simulink model "Main_simulation_optimised_accel_testbed"  (R2017b)
settings: Solver=FixedStepDiscrete  StartTime=0  StopTime=2474  RelTol=1e-3  EnableMultiTasking=on
PreLoadFcn:
  | Ts=2e-6;
undefined symbols (not defined in the file): Batt, BatteryCback, BatteryLoadFcn, DiscIntNeverNeededParam, Discrete, gcbh, Ion, Lithium, sigbuilder_block, sps_rtmsupport, spsBatteryModel
libraries: powerlib x53, electricdrivelib x6, simulink x6, autolibshared x6, powerlib_meascontrol x4, sdolib x3, spsDrivesDcBusModel x1, spsDrivesPrivateModels x1, spsDrivesOutputSelector x1, spsDrivesSpeedControllerModel x1
(part 2 of 3)

== system Main_simulation_optimised_accel_testbed/PMSM Drive vehicle ==
  Speed (rad/sec) : Inport
  Trq (Nm) : Inport  Port=2
  Bus Creator : BusCreator  Inputs=3
  Bus Selector : BusSelector  OutputSignals=V bus (V)
  DC_bus overvoltage protection : Subsystem  Commented=on
  PM Synchronous Motor Drive : Subsystem  DialogController=POWERSYS.PowerSysDialog  LoadFcn=|  mask(PM Synchronous Motor Drive){Rs=0.2, Lls=8.5e-3, Lms=8.5e-3, MachineConstant=Flux linkage established by magnets (V.s), FluxCst=0.175, VoltageCst=126.966, TorqueCst=1.05, ia=0, ib=0, J=0.089, Friction=0.005, p=4, wm=0, thetam=0, Rsnb_rec=10e3, Csnb_rec=20e-9, Ron_rec=1e-3, Vf_rec=1.3, cap_bus=200e-6, Rbrake=8, fbrake=4000, activationVoltage=190, shutdownVoltage=175, sourceFrequency=60, deviceType=IGBT / Diodes, Ron_inv=1e-3, Vf_inv=0.8, Vfd_inv=0.8, Tf=1e-6, Tt=2e-6, Tf_GTO=0, Tt_GTO=0, Rsnb_inv=5000, Csnb_inv=inf, regulationType=Speed regulation, Acc=1000, Dec=-1000, kp_sc=5, ki_sc=100, fc_sc=100, Tsc=7*20e-6, Tmin=-17.8, Tmax=17.8, modulationType=Hysteresis, h=0.1, kp_Id=200, ki_Id=1000, kp_Iq=200, ki_Iq=1000, fc_bus=50, car_freq=20000, freq_max=20e3, Tvect=20e-6, baseSampleTime=2e-06, outputBusMode=Multiple output buses, busLabels=off, MechanicalLoad=Torque Tm, modelDetailLevel=Detailed, driveType=AC6, AverageValue=off}
      | if ~isempty(get_param(gcb,'UserData')) 
      |       UserDataToSimulinkMask(gcbh,get_param(gcb,'driveType'));  
      |       set_param(gcb, 'UserData',[]);
      |       set_param(gcb,'UserDataPersistent','off');
      | end 
      | if strcmp(get_param(gcb,'AverageValue'),'on')
      |     set_param(gcb,'modelDetailLevel','Average');
      | end
      mask prompts: Rs "Resistance (ohm):"; Lls "D-axis inductance (H):"; Lms "Q-axis inductance (H):"; MachineConstant "Specify:"; ia "Phase A (A):"; ib "Phase B (A):"; J "Inertia (kg.m^2):"; Friction "Friction factor (N.m.s):"; p "Pole pairs:"; wm "Speed (rad/s):"; thetam "Angle (deg):"; Rsnb_rec "Resistance (ohm):"; Csnb_rec "Capacitance (F):"; Ron_rec "On-state resistance (ohm):"; Vf_rec "Forward voltage (V):"; cap_bus "Capacitance (F):"; Rbrake "Resistance (ohm):"; fbrake "Chopper frequency (Hz):"; activationVoltage "Activation voltage (V):"; shutdownVoltage "Shutdown voltage (V):"; sourceFrequency "Source frequency (Hz):"; deviceType "Device type:"; Ron_inv "On-state resistance (ohm):"; Vf_inv "Main device:"; Vfd_inv "Diode:"; Tf "Fall time (s):"; Tt "Tail time (s):"; Tf_GTO "Fall time (s):"; Tt_GTO "Tail time (s):"; Rsnb_inv "Resistance (ohm):"; Csnb_inv "Capacitance (F):"; regulationType "Regulation type:"; Acc "Acceleration:"; Dec "Deceleration:"; kp_sc "Proportional gain:"; ki_sc "Integral gain:"; fc_sc "Speed cutoff frequency (Hz):"; Tsc "Speed controller sampling time (s):"; Tmin "Negative:"; Tmax "Positive:"; modulationType "Modulation type:"; h "Current controller hysteresis bandwidth (A):"; kp_Id "Proportional gain:"; ki_Id "Integral gain:"; kp_Iq "Proportional gain:"; ki_Iq "Integral gain:"; fc_bus "DC bus voltage sensor cutoff frequency (Hz):"; car_freq "SVM switching frequency (Hz):"; freq_max "Maximum  switching frequency (Hz):"; Tvect "Controller sampling time (s):"; baseSampleTime "Base sample time:"; outputBusMode "Output bus mode:"; busLabels "Use bus labels"; MechanicalLoad "Mechanical input:"; modelDetailLevel "Model detail level:"; driveType "Drive type:"; AverageValue "Average value model"
      mask help: Implements a classical vector control drive for permanent synchronous motors.
      mask init:
      | [X1,X1m,X2,X2m,X3,X4,Y1,Y1m,Y2,Y2m,Y3,Y4,color1,color2,INp,OUTp,machineType,baseSampleTime] = spsDrivesMaskInit(gcb,driveType,AverageValue);
      settings: OpenFcn=sps_rtmsupport('OpenFcn',gcbh)
      mask Help: helpview(psbhelp)
      mask TypeOptions MachineConstant: Flux linkage established by magnets (V.s) | Voltage Constant (V_peak L-L / krpm) | Torque Constant (N.m / A_peak)
      mask Callback MachineConstant:
      | block = gcb;
      | MC = get_param(block,'MachineConstant');
      | set_param([block,'/','Permanent Magnet Synchronous Machine'],'MachineConstant',MC);
      | set_param([block,'/','VECT'],'MachineConstant',MC);
      | switch MC
      |     case 'Flux linkage established by magnets (V.s)'
      |         set_param([block,'/','Permanent Magnet Synchronous Machine'],'Flux',get_param(block,'FluxCst'))
      |     case 'Voltage Constant (V_peak L-L / krpm)'
      |         set_param([block,'/','Permanent Magnet Synchronous Machine'],'VoltageCst',get_param(block,'VoltageCst'))
      |     case 'Torque Constant (N.m / A_peak)'
      |         set_param([block,'/','Permanent Magnet Synchronous Machine'],'TorqueCst',get_param(block,'TorqueCst'))
      | end
      mask Callback FluxCst:
      | block = gcb;
      | MC = get_param(block,'MachineConstant');
      | set_param([block,'/','Permanent Magnet Synchronous Machine'],'MachineConstant',MC);
      | set_param([block,'/','VECT'],'MachineConstant',MC);
      | switch MC
      |     case 'Flux linkage established by magnets (V.s)'
      |         set_param([block,'/','Permanent Magnet Synchronous Machine'],'Flux',get_param(block,'FluxCst'))
      |     case 'Voltage Constant (V_peak L-L / krpm)'
      |         set_param([block,'/','Permanent Magnet Synchronous Machine'],'VoltageCst',get_param(block,'VoltageCst'))
      |     case 'Torque Constant (N.m / A_peak)'
      |         set_param([block,'/','Permanent Magnet Synchronous Machine'],'TorqueCst',get_param(block,'TorqueCst'))
      | end
      mask Callback VoltageCst:
      | block = gcb;
      | MC = get_param(block,'MachineConstant');
      | set_param([block,'/','Permanent Magnet Synchronous Machine'],'MachineConstant',MC);
      | set_param([block,'/','VECT'],'MachineConstant',MC);
      | switch MC
      |     case 'Flux linkage established by magnets (V.s)'
      |         set_param([block,'/','Permanent Magnet Synchronous Machine'],'Flux',get_param(block,'FluxCst'))
      |     case 'Voltage Constant (V_peak L-L / krpm)'
      |         set_param([block,'/','Permanent Magnet Synchronous Machine'],'VoltageCst',get_param(block,'VoltageCst'))
      |     case 'Torque Constant (N.m / A_peak)'
      |         set_param([block,'/','Permanent Magnet Synchronous Machine'],'TorqueCst',get_param(block,'TorqueCst'))
      | end
      mask Callback TorqueCst:
      | block = gcb;
      | MC = get_param(block,'MachineConstant');
      | set_param([block,'/','Permanent Magnet Synchronous Machine'],'MachineConstant',MC);
      | set_param([block,'/','VECT'],'MachineConstant',MC);
      | switch MC
      |     case 'Flux linkage established by magnets (V.s)'
      |         set_param([block,'/','Permanent Magnet Synchronous Machine'],'Flux',get_param(block,'FluxCst'))
      |     case 'Voltage Constant (V_peak L-L / krpm)'
      |         set_param([block,'/','Permanent Magnet Synchronous Machine'],'VoltageCst',get_param(block,'VoltageCst'))
      |     case 'Torque Constant (N.m / A_peak)'
      |         set_param([block,'/','Permanent Magnet Synchronous Machine'],'TorqueCst',get_param(block,'TorqueCst'))
      | end
      mask TypeOptions deviceType: GTO / Diodes | MOSFET / Diodes | IGBT / Diodes
      mask Callback deviceType: set_param([gcb,'/Three-phase Inverter'],'Device',get_param(gcb,'deviceType'));
      mask TypeOptions regulationType: Speed regulation | Torque regulation
      mask Callback regulationType: set_param([gcb '/Speed Controller'],'SwK',get_param(gcb,'regulationType'));
      mask TypeOptions modulationType: Hysteresis | SVM
      mask TypeOptions outputBusMode: Multiple output buses | Single output bus
      mask TypeOptions MechanicalLoad: Torque Tm | Speed w | Mechanical rotational port
      mask TypeOptions modelDetailLevel: Detailed | Average
      mask Callback modelDetailLevel:
      | if strcmp(get_param(gcb,'modelDetailLevel'),'Average')
      |    set_param(gcb,'AverageValue','on');
      | else
      |    set_param(gcb,'AverageValue','off');
      | end
      mask TypeOptions driveType: AC6
      mask DialogControl Container7 Prompt: Permanent Magnet Synchronous Machine
      mask DialogControl Container22 Prompt: Electrical parameters
      mask DialogControl Container27 Prompt: Equivalent circuit parameters
      mask DialogControl Container21 Prompt: Flux constant
      mask DialogControl Container34 Prompt: Initial currents
      mask DialogControl Container23 Prompt: Mechanical parameters
      mask DialogControl Container36 Prompt: Initial  values
      mask DialogControl Container10 Prompt: Converters and DC bus
      mask DialogControl Container28 Prompt: Rectifier
      mask DialogControl Container26 Prompt: Snubbers
      mask DialogControl Container29 Prompt: Diodes
      mask DialogControl Container30 Prompt: DC bus
      mask DialogControl Container31 Prompt: Braking chopper
      mask DialogControl Container32 Prompt: Inverter
      mask DialogControl Container37 Prompt: Switches
      mask DialogControl Forwardvoltages Prompt: Forward voltages (V)
      mask DialogControl Turnoff Prompt: Turn-off characteristics
      mask DialogControl InvSnubbers Prompt: Snubbers
      mask DialogControl Container12 Prompt: Controller
      mask DialogControl Control5 Prompt: Schematic
      mask DialogControl Control5 Callback:
      | openfig('ac6.fig','invisible');
      | movegui(gcf,'northwest');
      | set(gcf,'Visible','on');
      mask DialogControl Container33 Prompt: Speed controller
      mask DialogControl Speedramp Prompt: Speed ramps (rpm/s)
      mask DialogControl PIregulator Prompt: PI regulator
      mask DialogControl Container43 Prompt: Torque output limits (N.m)
      mask DialogControl Container35 Prompt: Vector control
      mask DialogControl d_axiscurrentregulator Prompt: d-axis current regulator
      mask DialogControl q_axiscurrentregulator Prompt: q-axis current regulator
      mask DialogControl Container47 Prompt: Parameters file options
      mask DialogControl Control3 Prompt: Load
      mask DialogControl Control3 Callback: loadValues(gcb,get_param(gcb,'driveType'));
      mask DialogControl Control4 Prompt: Save
      mask DialogControl Control4 Callback: saveValues(gcb,get_param(gcb,'driveType'));
      mask Display:
      | patch([X1 X1m],[Y1 Y1m],color1);
      | patch(X3,Y3,color2);
      | plot([X1 X1m X2 X2m X3 X4],[Y1 Y1m Y2 Y2m Y3 Y4]);
      | text(0.5,0.3,'AC6','HorizontalAlignment','center')
      | HaveSPSMec = (strcmp(MechanicalLoad,'Torque Tm') || strcmp(MechanicalLoad,'Speed w'));
      | color('blue');
      | if (HaveSPSMec==1 && strcmp(outputBusMode,'Multiple output buses'))
      |     port_label('input',2,INp)
      |     port_label('output',4,OUTp)
      | end
      | if (HaveSPSMec==1 && strcmp(outputBusMode,'Single output bus'))
      |     port_label('input',2,INp)
      |     port_label('output',2,OUTp)
      | end
  PM Synchronous Motor Drive1 : electricdrivelib/AC drives/PM Synchronous Motor Drive  Commented=on  Rs=0.2  Lls=8.5e-3  Lms=8.5e-3  MachineConstant=Flux linkage established by magnets (V.s)  FluxCst=0.175  VoltageCst=126.966  TorqueCst=1.05  ia=0  ib=0  J=0.089  Friction=0.005  p=4  wm=0  thetam=0  Rsnb_rec=10e3  Csnb_rec=20e-9  Ron_rec=1e-3  Vf_rec=1.3  cap_bus=2000e-6  Rbrake=8  fbrake=4000  activationVoltage=320  shutdownVoltage=310  sourceFrequency=60  deviceType=IGBT / Diodes  Ron_inv=1e-3  Vf_inv=0.8  Vfd_inv=0.8  Tf=1e-6  Tt=2e-6  Tf_GTO=0  Tt_GTO=0  Rsnb_inv=5000  Csnb_inv=inf  regulationType=Speed regulation  Acc=1000  Dec=-1000  kp_sc=5  ki_sc=100  fc_sc=100  Tsc=7*20e-6  Tmin=-17.8  Tmax=17.8  modulationType=Hysteresis  h=0.1  kp_Id=200  ki_Id=1000  kp_Iq=200  ki_Iq=1000  fc_bus=50  car_freq=20000  freq_max=20e3  Tvect=20e-6  baseSampleTime=2e-06  outputBusMode=Multiple output buses  busLabels=off  MechanicalLoad=Torque Tm  modelDetailLevel=Detailed  driveType=AC6  AverageValue=off
      link override VECT: machineConstant=Flux linkage established by magnets (V.s)
      settings: SourceProductName=Simscape Power Systems  SourceProductBaseCode=PS
  + : PMIOPort  Port=1  Side=Left
  - : PMIOPort  Port=2  Side=Left
  wm : Outport
  Feedback : Outport  Port=2
  wires:
  PM Synchronous Motor Drive/3(Ctrl) -> Bus Creator/3
  PM Synchronous Motor Drive/2(Conv.) -> Bus Selector/1, Bus Creator/2
  PM Synchronous Motor Drive/1(Motor) -> Bus Creator/1
  PM Synchronous Motor Drive/4(Wm) -> wm/1
  Bus Creator/1 -> Feedback/1
  Bus Selector/1 -> DC_bus overvoltage protection/1(DC_Bus_Voltage)  "<V bus (V)>"
  Speed (rad/sec)/1 -> PM Synchronous Motor Drive/1(SP)
  Trq (Nm)/1 -> PM Synchronous Motor Drive/2(Tm)
  connections:
  PM Synchronous Motor Drive/LConn1 -- DC_bus overvoltage protection/LConn1 -- +/RConn1
  PM Synchronous Motor Drive/LConn2 -- DC_bus overvoltage protection/LConn2 -- -/RConn1

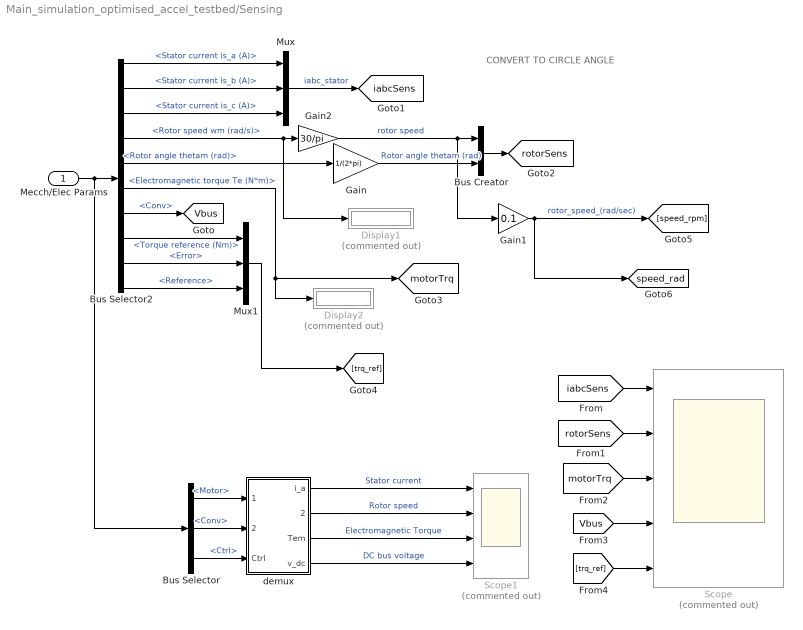
== system Main_simulation_optimised_accel_testbed/Sensing ==
  note: CONVERT TO CIRCLE ANGLE
  Mecch/Elec Params : Inport
  Bus Creator : BusCreator  Inputs=2
  Bus Selector : BusSelector  OutputSignals=Motor,Conv,Ctrl
  Bus Selector2 : BusSelector  OutputSignals=Motor.Stator current is_a (A),Motor.Stator current is_b (A),Motor.Stator current is_c (A),Motor.Rotor speed wm (rad/s),Motor.Rotor angle thetam (rad),Motor.Electromagnetic torque Te (N*m),Conv,Ctrl.Torque reference (Nm),Ctrl.Error,Ctrl.Reference
  Display1 : Display  Commented=on
  Display2 : Display  Commented=on
  Gain : Gain  Gain=1/(2*pi)
  Gain1 : Gain  Gain=0.1
  Gain2 : Gain  Gain=30/pi  SaturateOnIntegerOverflow=on  OutDataTypeStr=Inherit: Same as input  ParamDataTypeStr=Inherit: Same as input
  Mux : Mux  Inputs=3
  Mux1 : Mux  Inputs=3
  Scope : Scope  Commented=on  NumInputPorts=5
  Scope1 : Scope  Commented=on  NumInputPorts=4
  demux : Subsystem
  tag scope: Vbus=global, iabcSens=global, motorTrq=global, rotorSens=global, speed_rad=global
  wires:
  Bus Selector2/5 -> Gain/1  "<Rotor angle thetam (rad)>"
  Mux/1 -> [iabcSens]  "iabc_stator"
  Bus Selector2/3 -> Mux/3  "<Stator current is_c (A)>"
  Mecch/Elec Params/1 -> Bus Selector/1, Bus Selector2/1
  Bus Creator/1 -> [rotorSens]
  Bus Selector2/4 -> Display1/1, Gain2/1  "<Rotor speed wm (rad/s)>"
  Bus Selector2/1 -> Mux/1  "<Stator current is_a (A)>"
  Bus Selector2/2 -> Mux/2  "<Stator current is_b (A)>"
  Bus Selector2/6 -> [motorTrq], Display2/1  "<Electromagnetic torque Te (N*m)>"
  Gain/1 -> Bus Creator/2  "Rotor angle thetam (rad)"
  Bus Selector2/7 -> [Vbus]  "<Conv>"
  Bus Selector2/8 -> Mux1/1  "<Torque reference (Nm)>"
  Bus Selector2/9 -> Mux1/2  "<Error>"
  Bus Selector2/10 -> Mux1/3  "<Reference>"
  Mux1/1 -> [trq_ref]
  [iabcSens] -> Scope/1
  [rotorSens] -> Scope/2
  [motorTrq] -> Scope/3
  [Vbus] -> Scope/4
  [trq_ref] -> Scope/5
  Gain1/1 -> [speed_rad], [speed_rpm]  "rotor_speed_(rad/sec)"
  demux/2(speed) -> Scope1/2  "Rotor speed"
  demux/1(i_a) -> Scope1/1  "Stator current"
  Bus Selector/1 -> demux/1(motor)  "<Motor>"
  Bus Selector/2 -> demux/2(Conv.)  "<Conv>"
  demux/4(v_dc) -> Scope1/4  "DC bus voltage"
  demux/3(Tem) -> Scope1/3  "Electromagnetic Torque"
  Bus Selector/3 -> demux/3(Ctrl)  "<Ctrl>"
  Gain2/1 -> Gain1/1, Bus Creator/1  "rotor speed"

== system Main_simulation_optimised_accel_testbed/Speed and Cooling  ==
  note: -exp(0.1*v/10)
  note: to generate speed based cooling rate
  note: not consiidering drag to keep it linear
  note: Y (kmph) = X(r/s) * 100 (kmph) / 400 (r/s)
  Gain1 : Gain  Gain=0.1/10
  Gain2 : Gain  Gain=100/400
  Math Function : Math  SaturateOnIntegerOverflow=on
  cooling_rate : Gain  Gain=-1
  tag scope: cooling_rate=global
  wires:
  Math Function/1 -> cooling_rate/1
  Gain1/1 -> Math Function/1
  [speed_rad] -> Gain2/1
  Gain2/1 -> Gain1/1
  cooling_rate/1 -> [cooling_rate]

== system Main_simulation_optimised_accel_testbed/Speed ref2 ==
  Demux : Demux  Tag=STV Demux  Outputs=1
  FromWs : FromWorkspace  Tag=STV FromWs  VariableName=tuvar  SampleTime=0
      SigBuilderData=|
      | common.afterFinalStr = 'Extrapolate'
      | common.sampleTime = 0
      | dataSet.timeRange = [0 20]
      | dataSet.name = 'Group 1'
      | sbobj.Groups.Name = 'Group 1'
      | sbobj.Groups.Signals.Name = 'Speed_Reference'
      | sbobj.Groups.Signals.XData = [0 1 1 2 2 2.39 2.39 3.81 5 5 6.45 6.48 6.8 7 8 8.05 9 9.1 10.2 11.4 11.58 12.5 13 13.46 14 14.26 14.48 15.04 15.2 15.4 15.5 15.64 17 18.1 18.42 18.74 19.3 19.52 20]
      | sbobj.Groups.Signals.YData = [0 5.1 0.2 11 7.5 2.4 0.6 7.1 1.2 0.4 8.7 8.1 15.3 13.2 12.9 11.3 7.1 2 2 9.26428571429 8.9 11.2014285714 16.7 17.2 10.45 11.9709897611 14.3 13.8 9.8 11.95 11.2641638225 12.65 12.65 6.4 0 0 1.3 0 0]
      | sbobj.Groups.TimeRange = [0 20]
  Speed_Reference : Outport  Tag=STV Outport
  wires:
  FromWs/1 -> Demux/1
  Demux/1 -> Speed_Reference/1

== system Main_simulation_optimised_accel_testbed/Temperature ==
  note: BATTERY TEMPERATURE
  Bus Creator : BusCreator  Commented=on  Inputs=2
  Constant : Constant  Value=2
  From3 : From  Commented=on  GotoTag=motor_temp  TagVisibility=global
  From4 : From  Commented=on  GotoTag=batt_temp  TagVisibility=global
  Gain1 : Gain  Gain=0.6
  Goto2 : Goto  Commented=on  GotoTag=temp  TagVisibility=global
  Mean : powerlib_meascontrol/Measurements/Mean  Commented=on  Freq=300  Vinit=30  Ts=0
  Motor_Temp_Subsys : Subsystem  Commented=on
  Saturation : Saturate  UpperLimit=48  LowerLimit=20
  Saturation1 : Saturate  UpperLimit=0  LowerLimit=-20
  Scope : Scope  Commented=on  NumInputPorts=2
  Subtract : Sum  Inputs=+++-
  Terminator : Terminator
  passive : Constant  Value=10
  tag scope: batt_temp=global
  wires:
  Subtract/1 -> Saturation/1
  passive/1 -> Subtract/4
  Saturation1/1 -> Subtract/3
  [cooling_rate] -> Saturation1/1
  Saturation/1 -> [batt_temp], Scope/2  "batt_temp(C)"
  [batt_curr] -> Gain1/1
  Gain1/1 -> Subtract/2
  From3/1 -> Bus Creator/1
  From4/1 -> Bus Creator/2
  Bus Creator/1 -> Goto2/1
  Mean/1 -> ?
  Constant/1 -> Terminator/1
  [temp_amb] -> Subtract/1
  Motor_Temp_Subsys/1(Out1) -> [temp_amb]
  Motor_Temp_Subsys/2(motor_temp(C)) -> Scope/1

== system Main_simulation_optimised_accel_testbed/Torque Ref ==
  Demux : Demux  Tag=STV Demux  Outputs=1
  FromWs : FromWorkspace  Tag=STV FromWs  VariableName=tuvar  SampleTime=0
      SigBuilderData=|
      | common.afterFinalStr = 'Extrapolate'
      | common.sampleTime = 0
      | dataSet.timeRange = [0 20]
      | dataSet.name = 'Group 1'
      | sbobj.Groups.Name = 'Group 1'
      | sbobj.Groups.Signals.Name = 'Signal 2'
      | sbobj.Groups.Signals.XData = [0 1 1.3 2 2 2.39 2.39 3.81 4.29 4.6 6.1 6.45 6.55 6.55 8 9 9.4 10 20]
      | sbobj.Groups.Signals.YData = [2.05 9.95 -8.5 13.8 -5 6.5 -5.2 7 -8.4 -1.3 8.7 -4.1 14.7 -1.9 11.6 11.5 -5.3 0 0]
      | sbobj.Groups.TimeRange = [0 20]
  Signal 2 : Outport  Tag=STV Outport
  wires:
  Demux/1 -> Signal 2/1
  FromWs/1 -> Demux/1

== system Main_simulation_optimised_accel_testbed/UCC_MCC_scopes  ==
  Bus Selector1 : BusSelector  OutputSignals=I_hv,Vhv,Ilv,Vlv
  Bus Selector2 : BusSelector  OutputSignals=meas_dcdc_bb_conv,Ultracapacitor_current <A>,Ultra Capacitor Voltage <V>
  From2 : From  Commented=on  GotoTag=switch_sig  TagVisibility=global
  From43 : From  Commented=on  GotoTag=mcc_sw  TagVisibility=global
  Scope7 : Scope  Commented=on  NumInputPorts=2
  Scope8 : Scope  NumInputPorts=3
  Scope9 : Scope  NumInputPorts=4
  wires:
  Bus Selector1/3 -> Scope9/3  "<Ilv>"
  Bus Selector2/1 -> Scope8/1  "<meas_dcdc_bb_conv>"
  [UCS_meas] -> Bus Selector2/1
  Bus Selector1/2 -> Scope9/2  "<Vhv>"
  Bus Selector1/1 -> Scope9/1  "<I_hv>"
  Bus Selector1/4 -> Scope9/4  "<Vlv>"
  [BiDC_IO_VImeas] -> Bus Selector1/1
  Bus Selector2/2 -> Scope8/2  "<Ultracapacitor_current <A>>"
  From43/1 -> Scope7/1  "mcc_sw_0B1C"
  Bus Selector2/3 -> Scope8/3  "<Ultra Capacitor Voltage <V>>"
  From2/1 -> Scope7/2  "BiDC control"

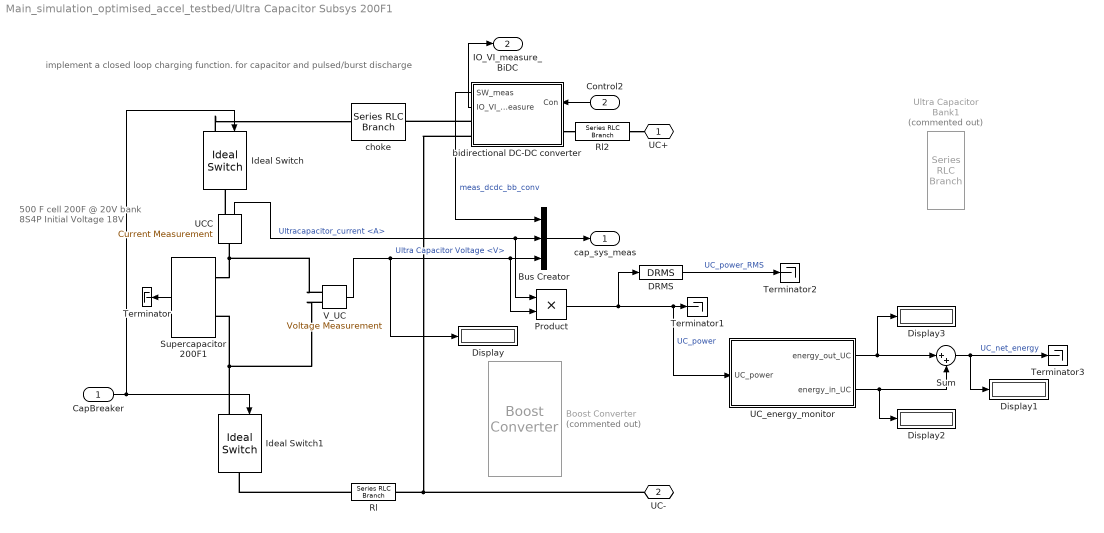
== system Main_simulation_optimised_accel_testbed/Ultra Capacitor Subsys 200F1 ==
  note: 500 F cell
      |
      | 200F @ 20V bank
      | 8S4P
      |
      | Initial Voltage 18V
  note: implement a closed loop charging function. for capacitor and pulsed/burst discharge
  CapBreaker : Inport
  Control2 : Inport  Port=2
  Boost Converter : powerlib/Power Electronics/Boost Converter  Commented=on  ModelType=Switching devices  Ron=1e-3  Rs=1e6  Cs=inf  Vforward=[0,0]  Ron_Diode=1e-3  Rs_Diode=1e6  Cs_Diode=inf  Vf_Diode=1e-3  Rs_CurrentSource=inf
      settings: SourceProductName=Simscape Power Systems  SourceProductBaseCode=PS
  Bus Creator : BusCreator  Inputs=3
  DRMS : sdolib/RMS Blocks/DRMS  Ts=10e-6
      settings: SourceProductName=Simulink Design Optimization  SourceProductBaseCode=SO
  Display{,1..3} (4 alike) : Display
  Ideal Switch : powerlib/Power Electronics/Ideal Switch  Ron=0.001  Lon=0  IC=0  Rs=10e6  Cs=inf  Measurements=off
  Ideal Switch1 : powerlib/Power Electronics/Ideal Switch  Ron=0.001  Lon=0  IC=0  Rs=10e6  Cs=inf  Measurements=off
  Product : Product
  Rl : powerlib/Elements/Series RLC Branch  LConnTagsString=__new0  RConnTagsString=__new0  BranchType=R  Resistance=0.05  Inductance=10e-6  SetiL0=off  InitialCurrent=0  Capacitance=1e-6  Setx0=off  InitialVoltage=0  Measurements=None
  Rl2 : powerlib/Elements/Series RLC Branch  LConnTagsString=__new0  RConnTagsString=__new0  BranchType=R  Resistance=0.05  Inductance=10e-6  SetiL0=off  InitialCurrent=0  Capacitance=1e-6  Setx0=off  InitialVoltage=0  Measurements=None
  Sum : Sum  Inputs=|++
  Supercapacitor 200F1 : electricdrivelib/Extra Sources/Supercapacitor  C=200  Rdc=15e-3  Voltage=20  Ns=8  Np=4  Vinit=12  Temp=25  PresetModel=off  EstParam=off  Nc=1  r=1e-9  epsilon=6.0208e-10  Ich=10  Vstern="[0.161  2.7  7.8]"  Self_dis=off  Ioc=10  Vself="[48  47.8  47.06  44.65]"  demandeplot=off  I="[10  20 100  500]"  Units=sec  Vmax=0  If=0  deltaV=0  alpha=0  sec=0
      settings: SourceProductName=Simscape Power Systems  SourceProductBaseCode=PS
  Terminator{,1..3} (4 alike) : Terminator
  UCC : powerlib/Measurements/Current Measurement  PhasorSimulation=off  OutputType=Complex  PSBequivalent=0
  UC_energy_monitor : Subsystem
  Ultra Capacitor Bank1 : powerlib/Elements/Series RLC Branch  Commented=on  LConnTagsString=__new0  RConnTagsString=__new0  BranchType=RC  Resistance=0.04  Inductance=1e-3  SetiL0=off  InitialCurrent=0  Capacitance=200  Setx0=on  InitialVoltage=18  Measurements=None
  V_UC : powerlib/Measurements/Voltage Measurement  PhasorSimulation=off  OutputType=Complex  PSBequivalent=0
  bidirectional DC-DC converter : Subsystem
  choke : powerlib/Elements/Series RLC Branch  LConnTagsString=__new0  RConnTagsString=__new0  BranchType=RL  Resistance=0.01  Inductance=10e-6  SetiL0=off  InitialCurrent=0  Capacitance=1e-6  Setx0=off  InitialVoltage=0  Measurements=None
  UC+ : PMIOPort  Port=1  Side=Right
  UC- : PMIOPort  Port=2  Side=Right
  cap_sys_meas : Outport
  IO_VI_measure_BiDC : Outport  Port=2
  wires:
  CapBreaker/1 -> Ideal Switch1/1, Ideal Switch/1
  Control2/1 -> bidirectional DC-DC converter/1(Con)
  bidirectional DC-DC converter/1(SW_meas) -> Bus Creator/1  "meas_dcdc_bb_conv"
  Bus Creator/1 -> cap_sys_meas/1
  UCC/1 -> Product/1, Bus Creator/2  "Ultracapacitor_current <A>"
  V_UC/1 -> Display/1, Product/2, Bus Creator/3  "Ultra Capacitor Voltage <V>"
  bidirectional DC-DC converter/2(IO_VI_measure) -> IO_VI_measure_BiDC/1
  Supercapacitor 200F1/1 -> Terminator/1
  DRMS/1 -> Terminator2/1  "UC_power_RMS"
  Product/1 -> DRMS/1, UC_energy_monitor/1(UC_power), Terminator1/1  "UC_power"
  Sum/1 -> Display1/1, Terminator3/1  "UC_net_energy"
  UC_energy_monitor/1(energy_out_UC) -> Display3/1, Sum/1
  UC_energy_monitor/2(energy_in_UC) -> Display2/1, Sum/2
  connections:
  Ideal Switch1/LConn1 -- Supercapacitor 200F1/LConn2 -- V_UC/LConn2
  V_UC/LConn1 -- Supercapacitor 200F1/LConn1 -- UCC/LConn1
  Ideal Switch/LConn1 -- choke/LConn1
  UC-/RConn1 -- Rl/RConn1 -- bidirectional DC-DC converter/RConn2
  bidirectional DC-DC converter/RConn1 -- choke/RConn1
  Rl2/RConn1 -- UC+/RConn1
  UCC/RConn1 -- Ideal Switch/RConn1
  Rl/LConn1 -- Ideal Switch1/RConn1
  bidirectional DC-DC converter/LConn1 -- Rl2/LConn1

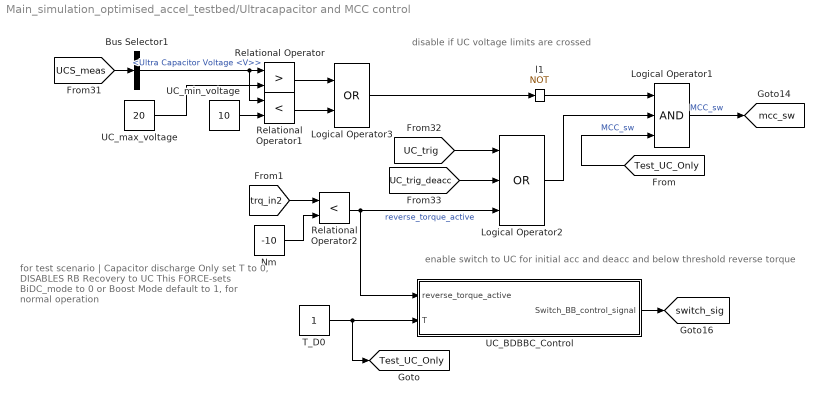
== system Main_simulation_optimised_accel_testbed/Ultracapacitor and MCC control ==
  note: enable switch to UC for initial acc and deacc and below threshold reverse torque
  note: disable if UC voltage limits are crossed
  note: for test scenario | Capacitor discharge Only
      | set T to 0,
      |
      | DISABLES RB Recovery to UC
      |
      | This FORCE-sets BiDC_mode to 0 or Boost Mode
      |
      | default to 1, for normal
      | operation
  Bus Selector1 : BusSelector  OutputSignals=Ultra Capacitor Voltage <V>
  Logical Operator1 : Logic  Inputs=3  AllPortsSameDT=off  OutDataTypeStr=boolean
  Logical Operator2 : Logic  Operator=OR  Inputs=3  AllPortsSameDT=off  OutDataTypeStr=boolean
  Logical Operator3 : Logic  Operator=OR  AllPortsSameDT=off  OutDataTypeStr=boolean
  Nm : Constant  Value=-10
  Relational Operator : RelationalOperator  Operator=>  OutDataTypeStr=boolean  RndMeth=Simplest
  Relational Operator1 : RelationalOperator  Operator=<  OutDataTypeStr=boolean  RndMeth=Simplest
  Relational Operator2 : RelationalOperator  Operator=<  OutDataTypeStr=boolean  RndMeth=Simplest
  T_D0 : Constant
  UC_BDBBC_Control : Subsystem
  UC_max_voltage : Constant  Value=20
  UC_min_voltage : Constant  Value=10
  l1 : Logic  Operator=NOT  IconShape=distinctive  AllPortsSameDT=off  OutDataTypeStr=boolean
  tag scope: Test_UC_Only=global, mcc_sw=global, switch_sig=global
  wires:
  UC_BDBBC_Control/1(Switch_BB_control_signal) -> [switch_sig]
  UC_min_voltage/1 -> Relational Operator1/2
  Relational Operator/1 -> Logical Operator3/1
  Relational Operator1/1 -> Logical Operator3/2
  Bus Selector1/1 -> Relational Operator1/1, Relational Operator/1  "<Ultra Capacitor Voltage <V>>"
  UC_max_voltage/1 -> Relational Operator/2
  Logical Operator3/1 -> l1/1
  Logical Operator2/1 -> Logical Operator1/2
  [UC_trig] -> Logical Operator2/1
  [UCS_meas] -> Bus Selector1/1
  l1/1 -> Logical Operator1/1
  Logical Operator1/1 -> [mcc_sw]  "MCC_sw"
  [UC_trig_deacc] -> Logical Operator2/2
  [trq_in2] -> Relational Operator2/1
  Nm/1 -> Relational Operator2/2
  Relational Operator2/1 -> UC_BDBBC_Control/1(reverse_torque_active), Logical Operator2/3  "reverse_torque_active"
  [Test_UC_Only] -> Logical Operator1/3  "MCC_sw"
  T_D0/1 -> [Test_UC_Only], UC_BDBBC_Control/2(T)

== system Main_simulation_optimised_accel_testbed/Velocity_profile selector ==
  Bus Creator : BusCreator  Inputs=6
  Bus Selector : BusSelector  OutputSignals=FTP75
  Drive Cycle Source : autolibshared/Drive Cycle Source  Commented=on  cycleVar=IM240  tfinal="240  seconds"  cycleRepeat=off  outAccPort=off  t_wot1=5  xdot_woto=0  xdot_wot1=30  t_wot2=20  xdot_wot2=0  t_wotend=30  srcUnit=m/s  outUnit=m/s  srcAccUnit=m/s/s  outAccUnit=m/s^2  dt=100e-6
      settings: SourceProductName=Powertrain Blockset  SourceProductBaseCode=PW
  Drive Cycle Source1 : autolibshared/Drive Cycle Source  Commented=on  cycleVar=NYCC  tfinal="598  seconds"  cycleRepeat=off  outAccPort=off  t_wot1=5  xdot_woto=0  xdot_wot1=30  t_wot2=20  xdot_wot2=0  t_wotend=30  srcUnit=m/s  outUnit=m/s  srcAccUnit=m/s/s  outAccUnit=m/s^2  dt=100e-6
      settings: SourceProductName=Powertrain Blockset  SourceProductBaseCode=PW
  Drive Cycle Source2 : autolibshared/Drive Cycle Source  Commented=on  cycleVar=FTP75  tfinal="2474  seconds"  cycleRepeat=off  outAccPort=off  t_wot1=5  xdot_woto=0  xdot_wot1=30  t_wot2=20  xdot_wot2=0  t_wotend=30  srcUnit=m/s  outUnit=m/s  srcAccUnit=m/s/s  outAccUnit=m/s^2  dt=100e-6
      settings: SourceProductName=Powertrain Blockset  SourceProductBaseCode=PW
  Drive Cycle Source3 : autolibshared/Drive Cycle Source  Commented=on  cycleVar=FTP75  tfinal="2474  seconds"  cycleRepeat=off  outAccPort=off  t_wot1=5  xdot_woto=0  xdot_wot1=30  t_wot2=20  xdot_wot2=0  t_wotend=30  srcUnit=m/s  outUnit=m/s  srcAccUnit=m/s/s  outAccUnit=m/s^2  dt=100e-6
      settings: SourceProductName=Powertrain Blockset  SourceProductBaseCode=PW
  Drive Cycle Source4 : autolibshared/Drive Cycle Source  Commented=on  cycleVar=Japanese 10 Mode  tfinal="135  seconds"  cycleRepeat=off  outAccPort=off  t_wot1=5  xdot_woto=0  xdot_wot1=30  t_wot2=20  xdot_wot2=0  t_wotend=30  srcUnit=m/s  outUnit=m/s  srcAccUnit=m/s/s  outAccUnit=m/s^2  dt=100e-6
      settings: SourceProductName=Powertrain Blockset  SourceProductBaseCode=PW
  Drive Cycle Source5 : autolibshared/Drive Cycle Source  cycleVar=FTP75  tfinal="2474  seconds"  cycleRepeat=off  outAccPort=off  t_wot1=5  xdot_woto=0  xdot_wot1=30  t_wot2=20  xdot_wot2=0  t_wotend=30  srcUnit=m/s  outUnit=m/s  srcAccUnit=m/s/s  outAccUnit=m/s^2  dt=100e-6
      settings: SourceProductName=Powertrain Blockset  SourceProductBaseCode=PW
  Gain : Gain
  Rate Transition : RateTransition
  Vel_reference_user : Outport
  wires:
  Rate Transition/1 -> Vel_reference_user/1  "Vel_reference_user"
  Drive Cycle Source/1 -> Bus Creator/5  "IM240 (240s)"
  Gain/1 -> Rate Transition/1
  Bus Selector/1 -> Gain/1  "<FTP75>"
  Drive Cycle Source1/1 -> Bus Creator/3  "NYCC (598s)"
  Drive Cycle Source2/1 -> Bus Creator/4  "CUEDC SPC240 (240s)"
  Bus Creator/1 -> Bus Selector/1
  Drive Cycle Source4/1 -> Bus Creator/1  "Jap10 (135s)"
  Drive Cycle Source3/1 -> Bus Creator/2  "BAC-Arterial Cycle (270s)"
  Drive Cycle Source5/1 -> Bus Creator/6  "FTP75"

== system Main_simulation_optimised_accel_testbed/Battery_subsys/BMS_protection ==
  note: disable switch to batt for UC trigger events
  note: disable if battery voltage limits are crossed
  Abs : Abs
  Batt_max_voltage<V> : Constant  Value=140
  Batt_min_voltage<V> : Constant  Value=110
  Derivative : Derivative
  Imax_batt_limit <A> pulse : Constant  Value=50
  Logical Operator1 : Logic  AllPortsSameDT=off  OutDataTypeStr=boolean
  Logical Operator2 : Logic  Operator=OR  AllPortsSameDT=off  OutDataTypeStr=boolean
  Logical Operator3 : Logic  Operator=OR  Inputs=3  AllPortsSameDT=off  OutDataTypeStr=boolean
  Relational Operator : RelationalOperator  Operator=>  OutDataTypeStr=boolean  RndMeth=Simplest
  Relational Operator1 : RelationalOperator  Operator=<  OutDataTypeStr=boolean  RndMeth=Simplest
  Relational Operator2 : RelationalOperator  Operator=>  OutDataTypeStr=boolean  RndMeth=Simplest
  l1 : Logic  Operator=NOT  IconShape=distinctive  AllPortsSameDT=off  OutDataTypeStr=boolean
  l2 : Logic  Operator=NOT  IconShape=distinctive  AllPortsSameDT=off  OutDataTypeStr=boolean
  tag scope: BMS_batt_sw=global
  wires:
  [Vbatt] -> Relational Operator1/1, Relational Operator/1
  Relational Operator2/1 -> Logical Operator3/1  "I_bound_thresh"
  Imax_batt_limit <A> pulse/1 -> Relational Operator2/2
  [Ibatt] -> Abs/1
  [UC_trig] -> Logical Operator2/1
  Batt_min_voltage<V>/1 -> Relational Operator1/2
  Logical Operator2/1 -> l2/1
  Logical Operator1/1 -> [BMS_batt_sw]  "BMS_relay"
  Relational Operator/1 -> Logical Operator3/2  "V_upper_thresh"
  [UC_trig_deacc] -> Logical Operator2/2
  l1/1 -> Logical Operator1/1
  Relational Operator1/1 -> Logical Operator3/3  "V_lower_thresh"
  Batt_max_voltage<V>/1 -> Relational Operator/2
  Logical Operator3/1 -> l1/1
  l2/1 -> Logical Operator1/2
  Derivative/1 -> Relational Operator2/1
  Abs/1 -> Derivative/1

== system Main_simulation_optimised_accel_testbed/Battery_subsys/BMS_relay ==
  Ideal Switch : powerlib/Power Electronics/Ideal Switch  Ron=0.001  Lon=0  IC=1  Rs=1e4  Cs=1e-8  Measurements=off
  Ideal Switch1 : powerlib/Power Electronics/Ideal Switch  Ron=0.001  Lon=0  IC=1  Rs=1e4  Cs=1e-8  Measurements=off
  L : powerlib/Elements/Series RLC Branch  LConnTagsString=__new0  RConnTagsString=__new0  BranchType=RL  Resistance=0.001  Inductance=20e-6  SetiL0=off  InitialCurrent=0  Capacitance=10e-6  Setx0=off  InitialVoltage=0  Measurements=None
  +Vo : PMIOPort  Port=1  Side=Right
  +B : PMIOPort  Port=2  Side=Left
  -Vo : PMIOPort  Port=3  Side=Right
  -B : PMIOPort  Port=4  Side=Left
  wires:
  [BMS_batt_sw] -> Ideal Switch/1, Ideal Switch1/1
  connections:
  Ideal Switch1/RConn1 -- -Vo/RConn1
  Ideal Switch1/LConn1 -- -B/RConn1
  Ideal Switch/LConn1 -- +B/RConn1
  L/LConn1 -- +Vo/RConn1
  Ideal Switch/RConn1 -- L/RConn1

== system Main_simulation_optimised_accel_testbed/Battery_subsys/bad_adaptive ==
  note: Internal Resistance
  Controlled Voltage Source : powerlib/Electrical Sources/Controlled Voltage Source  Initialize=on  Source_Type=AC  Amplitude=0  Phase=0  Frequency=0  Measurements=None
  Current Measurement : powerlib/Measurements/Current Measurement  PhasorSimulation=off  OutputType=Complex  PSBequivalent=0
  Model : Subsystem  AncestorBlock=spsBatteryModel/Discrete
  Series RLC Branch : powerlib/Elements/Series RLC Branch  LConnTagsString=__new0  RConnTagsString=__new0  BranchType=R  Resistance=Batt.R  Inductance=1e-3  SetiL0=off  InitialCurrent=0  Capacitance=1e-6  Setx0=off  InitialVoltage=0  Measurements=None
  Ta : Constant  Value=Batt.Ta
  + : PMIOPort  Tag=PMCPort  Port=1  Side=Left
  - : PMIOPort  Tag=PMCPort  Port=2  Side=Left
  m : Outport
  wires:
  Ta/1 -> Model/2(Ta)
  Current Measurement/1 -> Model/1(current)  "Current"
  Model/1(m) -> m/1
  Model/2(V) -> Controlled Voltage Source/1
  connections:
  Series RLC Branch/RConn1 -- Current Measurement/LConn1
  Controlled Voltage Source/RConn1 -- Series RLC Branch/LConn1
  Controlled Voltage Source/LConn1 -- -/RConn1
  +/RConn1 -- Current Measurement/RConn1

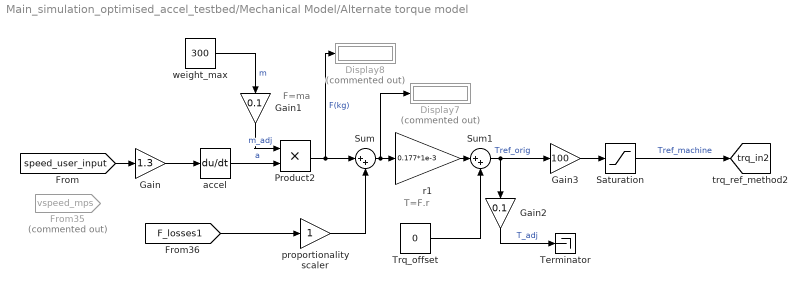
== system Main_simulation_optimised_accel_testbed/Mechanical Model/Alternate torque model ==
  note: T=F.r
  note: F=ma
  Display7 : Display  Commented=on
  Display8 : Display  Commented=on
  From35 : From  Commented=on  GotoTag=vspeed_mps  TagVisibility=global
  Gain : Gain  Gain=1.3
  Gain1 : Gain  Gain=0.1
  Gain2 : Gain  Gain=0.1
  Gain3 : Gain  Gain=100
  Product2 : Product
  Saturation : Saturate  UpperLimit=22  LowerLimit=-30
  Sum : Sum  Inputs=|++
  Sum1 : Sum  Inputs=|++
  Terminator : Terminator
  Trq_offset : Constant  Value=0
  accel : Derivative
  proportionality scaler : Gain
  r1 : Gain  Gain=0.177*1e-3
  weight_max : Constant  Value=300
  tag scope: trq_in2=global
  wires:
  weight_max/1 -> Gain1/1  "m"
  accel/1 -> Product2/2  "a"
  [speed_user_input] -> Gain/1
  [F_losses1] -> proportionality scaler/1
  Product2/1 -> Display8/1, Sum/1  "F(kg)"
  Sum1/1 -> Gain2/1, Gain3/1  "Tref_orig"
  Sum/1 -> Display7/1, r1/1
  r1/1 -> Sum1/1
  Trq_offset/1 -> Sum1/2
  Gain/1 -> accel/1
  proportionality scaler/1 -> Sum/2
  Gain1/1 -> Product2/1  "m_adj"
  Gain2/1 -> Terminator/1  "T_adj"
  Saturation/1 -> [trq_in2]  "Tref_machine"
  Gain3/1 -> Saturation/1

== system Main_simulation_optimised_accel_testbed/Mechanical Model/Gradient generator ==
  Demux : Demux  Tag=STV Demux  Outputs=1
  FromWs : FromWorkspace  Tag=STV FromWs  VariableName=tuvar  SampleTime=0
      SigBuilderData=|
      | common.afterFinalStr = 'Extrapolate'
      | common.sampleTime = 0
      | dataSet.timeRange = [0 10]
      | dataSet.name = 'Group 1'
      | sbobj.Groups.Name = 'Group 1'
      | sbobj.Groups.Signals.Name = 'Gradient'
      | sbobj.Groups.Signals.XData = [0 1 1.2 2.6 2.8 3.8 5 5.5 6.62 7.16 10]
      | sbobj.Groups.Signals.YData = [0 1 5 5 1.96 0.3 0.25 -2.2 -2.2 0 0]
  Gradient : Outport  Tag=STV Outport
  wires:
  FromWs/1 -> Demux/1
  Demux/1 -> Gradient/1

== system Main_simulation_optimised_accel_testbed/Mechanical Model/Signal Builder ==
  Demux : Demux  Tag=STV Demux  Outputs=1
  FromWs : FromWorkspace  Tag=STV FromWs  VariableName=tuvar  SampleTime=0
      SigBuilderData=|
      | common.afterFinalStr = 'Extrapolate'
      | common.sampleTime = 0
      | dataSet.timeRange = [0 10]
      | dataSet.name = 'Group 1'
      | sbobj.Groups.Name = 'Group 1'
      | sbobj.Groups.Signals.Name = 'Signal 2'
      | sbobj.Groups.Signals.XData = [0 1 1 2 2 2.39 2.39 3.81 5 5 6.45 6.45 6.8 6.8 8 8 9 9 10]
      | sbobj.Groups.Signals.YData = [0 5.1 0.2 11 7.5 2.4 0.6 7.1 1.2 0.4 8.7 7.7 14.7 13 13.2 11.3 7.1 0.2 0.2]
  Signal 2 : Outport  Tag=STV Outport
  wires:
  FromWs/1 -> Demux/1
  Demux/1 -> Signal 2/1

== system Main_simulation_optimised_accel_testbed/Mechanical Model/Torque model 1 -- redacted ==
  note: torque reference generation
  note: real torque gain factor - 0.1
      | for simulation - 0.01
  Abs : Abs
  Product1 : Product  Inputs=4
  Saturation1 : Saturate  UpperLimit=15  LowerLimit=-15
  Saturation2 : Saturate  UpperLimit=30  LowerLimit=-40
  torque gain : Constant  Value=5
  tag scope: torque_input=global
  wires:
  Saturation1/1 -> Product1/2
  Abs/1 -> Product1/3
  [acc_dec_rate] -> Saturation1/1
  Saturation2/1 -> [torque_input]  "trq_input"
  Product1/1 -> Saturation2/1
  torque gain/1 -> Product1/4
  [speed_ref] -> Product1/1
  [ad_detect] -> Abs/1

== system Main_simulation_optimised_accel_testbed/Mechanical Model/gradient generation ==
  Demux : Demux  Tag=STV Demux  Outputs=2
  FromWs : FromWorkspace  Tag=STV FromWs  VariableName=tuvar  SampleTime=0
      SigBuilderData=|
      | common.afterFinalStr = 'Extrapolate'
      | common.sampleTime = 0
      | dataSet.timeRange = [0 2475]
      | dataSet.name = 'Group 1'
      | sbobj.Groups.Name = 'Group 1'
      | sbobj.Groups.Signals(1).Name = 'HF_gradient'
      | sbobj.Groups.Signals(1).XData = [0 2 4 6 8 10 12 14 16 18 20 22 ... (1238 elements, 1x1238)]
      | sbobj.Groups.Signals(1).YData = [22.9417155399 3.79516890669 9.54455867252 2.11992787844 1.74272804988 6.01841469674 12.9877232925 5.85416125953 12.6883430705 11.8652937464 -16.0666412999 -0.88204602308 ... (1238 elements, 1x1238)]
      | sbobj.Groups.Signals(2).Name = 'LF_stable_gradient'
      | sbobj.Groups.Signals(2).XData = [0 30 50 124 200 328 500 1000 1398 1604 1800 2008 2112 2300 2475]
      | sbobj.Groups.Signals(2).YData = [1 0 10 7.8 -5 -5.8 0 0 4.8 4.8 2 -2.6 1 0 0]
      | sbobj.Groups.TimeRange = [0 2475]
  HF_gradient : Outport  Tag=STV Outport
  LF_stable_gradient : Outport  Tag=STV Outport  Port=2
  wires:
  FromWs/1 -> Demux/1
  Demux/1 -> HF_gradient/1
  Demux/2 -> LF_stable_gradient/1

== system Main_simulation_optimised_accel_testbed/Mechanical Model/scopes ==
  note: --------vehicle velocity
      |
      | --------drag1
      |
      | --------wind effect ( integrate into drag) - only for x-axis11
      |
      | ---------tire speed
      |
      | ---------torsional losses in axle
      |
      | ---------braking2
      |
      | ---------mechanical braking !!!!!!!!hold!
      |
      | ----------regen braking222
      |
      | ---------gradient effect3
      |
      | ----------gear box gain
  From14 : From  Commented=on  GotoTag=mtr_speed_ref  TagVisibility=global
  From15 : From  Commented=on  GotoTag=mtr_speed_ref_RPM  TagVisibility=global
  From16 : From  Commented=on  GotoTag=vspeed_mps  TagVisibility=global
  From17 : From  Commented=on  GotoTag=vspeed_kmph  TagVisibility=global
  From18 : From  Commented=on  GotoTag=Fd
  From19 : From  Commented=on  GotoTag=F_losses1  TagVisibility=global
  From20 : From  Commented=on  GotoTag=gradient
  From21 : From  Commented=on  GotoTag=act_wheel_drive_trq  TagVisibility=global
  From22 : From  Commented=on  GotoTag=torque_input  TagVisibility=global
  From23 : From  Commented=on  GotoTag=slope_detect  TagVisibility=global
  From24 : From  Commented=on  GotoTag=acc_dec_rate  TagVisibility=global
  From25 : From  Commented=on  GotoTag=mech_braking  TagVisibility=global
  From26 : From  Commented=on  GotoTag=UC_trig  TagVisibility=global
  From27 : From  Commented=on  GotoTag=torque_input  TagVisibility=global
  From28 : From  Commented=on  GotoTag=speed_input_drive
  Scope2 : Scope  Commented=on  NumInputPorts=9
  Scope3 : Scope  Commented=on  NumInputPorts=6
  wires:
  From28/1 -> Scope3/6
  From21/1 -> Scope2/8
  From14/1 -> Scope2/1
  From16/1 -> Scope2/3
  From17/1 -> Scope2/4
  From23/1 -> Scope3/1
  From20/1 -> Scope2/6
  From18/1 -> Scope2/5
  From22/1 -> Scope2/9
  From15/1 -> Scope2/2
  From27/1 -> Scope3/5
  From26/1 -> Scope3/4
  From25/1 -> Scope3/3
  From24/1 -> Scope3/2
  From19/1 -> Scope2/7

== system Main_simulation_optimised_accel_testbed/Mechanical Model/wind profile 2474 ==
  Demux : Demux  Tag=STV Demux  Outputs=1
  FromWs : FromWorkspace  Tag=STV FromWs  VariableName=tuvar  SampleTime=0
      SigBuilderData=|
      | common.afterFinalStr = 'Extrapolate'
      | common.sampleTime = 0
      | dataSet.timeRange = [0 2475]
      | dataSet.name = 'Group 1'
      | sbobj.Groups.Name = 'Group 1'
      | sbobj.Groups.Signals.Name = 'Wind_LF'
      | sbobj.Groups.Signals.XData = [0 100 200 300 400 500 600 700 800 900 1000 1100 1200 1300 1400 1500 1600 1700 1800 1900 2000 2100 2200 2300 2475]
      | sbobj.Groups.Signals.YData = [2.79319195475 0.482607832575 -2.35572767353 2.82051334745 0 0.1 -3.10818568071 3.1 2.3 0.705346289994 -5.69607660455 1.9 -1.45692010145 -2.25917814687 3.52742540056 -1.64483758534 -0.563905882684 -1.7 -4.81598219137 -5.42813591475 1.92501804763 -2.39839945129 2.8 1.9 0.838188322543]
      | sbobj.Groups.TimeRange = [0 2475]
  Wind_LF : Outport  Tag=STV Outport
  wires:
  FromWs/1 -> Demux/1
  Demux/1 -> Wind_LF/1

== system Main_simulation_optimised_accel_testbed/PMSM Drive vehicle/DC_bus overvoltage protection ==
  note: undervoltage and fault safety
  DC_Bus_Voltage : Inport
  Bleed load : powerlib/Elements/Series RLC Branch  LConnTagsString=__new0  RConnTagsString=__new0  BranchType=RL  Resistance=2  Inductance=5e-6  SetiL0=off  InitialCurrent=0  Capacitance=1e-6  Setx0=off  InitialVoltage=0  Measurements=None
  Bus_max_voltage<V> : Constant  Value=140
  Bus_min_voltage<V> : Constant  Value=108
  Ideal Switch : powerlib/Power Electronics/Ideal Switch  Ron=0.001  Lon=0  IC=0  Rs=10e3  Cs=1e-6  Measurements=off
  Logical Operator3 : Logic  Operator=OR  Inputs=3  AllPortsSameDT=off  OutDataTypeStr=boolean
  Relational Operator : RelationalOperator  Operator=>  OutDataTypeStr=boolean  RndMeth=Simplest
  Relational Operator1 : RelationalOperator  Operator=<  OutDataTypeStr=boolean  RndMeth=Simplest
  Relational Operator2 : RelationalOperator  Operator=>  OutDataTypeStr=boolean  RndMeth=Simplest
  A+ : PMIOPort  Port=1  Side=Left
  A- : PMIOPort  Port=2  Side=Left
  tag scope: disable_MCC=global
  wires:
  DC_Bus_Voltage/1 -> Relational Operator1/1, Relational Operator/1
  Relational Operator/1 -> Logical Operator3/3, Logical Operator3/2  "V_drive_upper_thresh"
  Bus_min_voltage<V>/1 -> Relational Operator1/2
  Logical Operator3/1 -> Ideal Switch/1  "over-voltage-DCbus"
  Bus_max_voltage<V>/1 -> Relational Operator2/2, Relational Operator/2
  [Vdc_bus_sfty] -> Relational Operator2/1
  Relational Operator2/1 -> Logical Operator3/1  "V_mcc_thresh"
  Relational Operator1/1 -> [disable_MCC]  "V_drive_lower_thresh"
  connections:
  Ideal Switch/RConn1 -- Bleed load/LConn1
  A+/RConn1 -- Ideal Switch/LConn1
  A-/RConn1 -- Bleed load/RConn1

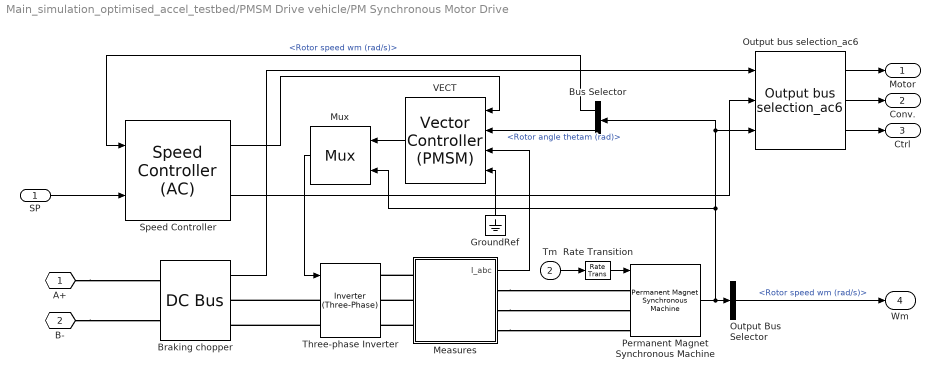
== system Main_simulation_optimised_accel_testbed/PMSM Drive vehicle/PM Synchronous Motor Drive ==
  SP : Inport
  Tm : Inport  Port=2
  Braking chopper : spsDrivesDcBusModel/DC Bus   busType=Capacitive (generic)  Ts=baseSampleTime  capacitance=cap_bus  inductance=0  Setx0=off  InitialVoltage=600  Rbrake=Rbrake  frequency=fbrake  activationVoltage=activationVoltage  shutdownVoltage=shutdownVoltage
      settings: SourceProductName=The database C:\Users\ak23510\AppData\Roaming\MathWorks\MATLAB\R2017a\slblocks_master.db is locked, or a table in the database is locked. (database is locked)
  Bus Selector : BusSelector  OutputSignals=Rotor speed wm (rad/s),Rotor angle thetam (rad)
  GroundRef : Ground
  Measures : Subsystem
  Mux : spsDrivesPrivateModels/Mux  OverrideUsingVariant=Detailed  detailLevel=Detailed  driveType=AC6
      settings: AttributesFormatString=%<BlockChoice>  SourceProductName=The database C:\Users\ak23510\AppData\Roaming\MathWorks\MATLAB\R2017a\slblocks_master.db is locked, or a table in the database is locked. (database is locked)
  Output Bus Selector : BusSelector  OutputSignals=Rotor speed wm (rad/s)
  Output bus selection_ac6 : spsDrivesOutputSelector/Output bus selection_ac6  OverrideUsingVariant=Multiple_output_buses
      settings: AttributesFormatString=%<BlockChoice>  SourceProductName=The database C:\Users\ak23510\AppData\Roaming\MathWorks\MATLAB\R2017a\slblocks_master.db is locked, or a table in the database is locked. (database is locked)
  Permanent Magnet Synchronous Machine : powerlib/Machines/Permanent Magnet Synchronous Machine  NbPhases=3  FluxDistribution=Sinusoidal  RotorType=Salient-pole  MechanicalLoad=Torque Tm  PresetModel=No  ShowDetailedParameters=on  MeasurementBus=off  Resistance=Rs  Inductance=0  dqInductances=[Lls,Lms]  La=0.000835  MachineConstant=Flux linkage established by magnets (V.s)  Flux=0.175  VoltageCst=126.966  TorqueCst=1.05  Flat=0  Mechanical=[J,Friction,p]  PolePairs=4  InitialConditions=[wm,thetam,ia,ib]  InitialConditions5ph=[0 0 0 0 0 0]  TsPowergui=0  TsBlock=-1  RefAngle=90 degrees behind phase A axis (modified Park)
      settings: AttributesFormatString=\n  SourceProductName=Simscape Power Systems
  Rate Transition : RateTransition  OutPortSampleTime=baseSampleTime
  Speed Controller : spsDrivesSpeedControllerModel/Speed Controller (AC)  OverrideUsingVariant=AC345  ctrlType=Without flux reference output  SwK=Speed regulation  Ts=baseSampleTime  ramp=[Dec,Acc]  kp=kp_sc  ki=ki_sc  fc=fc_sc  ctrl_sat=[Tmin,Tmax]  Tsc=Tsc  fn=60  p=2  nf=0.3
      settings: SourceProductName=The database C:\Users\ak23510\AppData\Roaming\MathWorks\MATLAB\R2017a\slblocks_master.db is locked, or a table in the database is locked. (database is locked)
  Three-phase Inverter : electricdrivelib/Fundamental Drive Blocks/Inverter (Three-Phase)  OverrideUsingVariant=Detailed  detailLevel=Detailed  driveType=PMSM vector control  Ts=baseSampleTime  SnubberResistance=Rsnb_inv  SnubberCapacitance=Csnb_inv  Device=IGBT / Diodes  Ron=Ron_inv  ForwardVoltages="[  Vf_inv  Vfd_inv  ]"  GTOparameters=[Tf_GTO,Tt_GTO]  IGBTparameters="[  Tf  Tt  ]"  Measurements=All voltages and currents  converterType=Inverter  SourceFrequency=sourceFrequency  ReferenceFrame=Rotor  dqInductances=[Lls,Lms]  Inductance=0  Ls=0  Resistance=Rs  Flux=FluxCst  Stator_sm=[2.01e-3,4.289e-4,4.477e-3,1.354e-3]  Stator_im=[14.85e-3,0.3027e-3]  Rotor=[9.295e-3,0.3027e-3]  Lm=10.46e-3  p=p
      settings: AttributesFormatString=%<BlockChoice>  SourceProductName=Simscape Power Systems  SourceProductBaseCode=PS
  VECT : electricdrivelib/Fundamental Drive Blocks/Vector Controller (PMSM)  OverrideUsingVariant=Detailed_3ph  detailLevel=Detailed  nb_ph=3  modulationType=Hysteresis  Ts_vect=Tvect  h=h  freq_max=freq_max  fc_bus=fc_bus  car_freq=car_freq  nb_p=p  machineConstant=Flux linkage established by magnets (V.s)  fluxConstant=FluxCst  voltageConstant=VoltageCst  torqueConstant=TorqueCst  kp_Id=kp_Id  ki_Id=ki_Id  kp_Iq=kp_Iq  ki_Iq=ki_Iq
      settings: AttributesFormatString=%<BlockChoice>  SourceProductName=Simscape Power Systems  SourceProductBaseCode=PS
  A+ : PMIOPort  Port=1  Side=Left
  B- : PMIOPort  Port=2  Side=Left
  Motor : Outport
  Conv. : Outport  Port=2
  Ctrl : Outport  Port=3
  Wm : Outport  Port=4
  wires:
  Mux/1 -> Three-phase Inverter/1
  Speed Controller/1 -> VECT/1
  Output bus selection_ac6/1 -> Motor/1
  Output bus selection_ac6/3 -> Ctrl/1
  Output bus selection_ac6/2 -> Conv./1
  Rate Transition/1 -> Permanent Magnet Synchronous Machine/1
  Tm/1 -> Rate Transition/1
  Output Bus Selector/1 -> Wm/1  "<Rotor speed wm (rad/s)>"
  Braking chopper/1 -> Output bus selection_ac6/1
  SP/1 -> Speed Controller/2
  Permanent Magnet Synchronous Machine/1 -> Output Bus Selector/1, Mux/2, Output bus selection_ac6/3, Bus Selector/1
  Measures/1(I_abc) -> VECT/3
  Speed Controller/2 -> Output bus selection_ac6/2
  VECT/1 -> Mux/1
  Bus Selector/1 -> Speed Controller/1  "<Rotor speed wm (rad/s)>"
  Bus Selector/2 -> VECT/2  "<Rotor angle thetam (rad)>"
  GroundRef/1 -> VECT/4
  connections:
  Three-phase Inverter/LConn2 -- Braking chopper/RConn2
  Three-phase Inverter/LConn1 -- Braking chopper/RConn1
  B-/RConn1 -- Braking chopper/LConn2
  A+/RConn1 -- Braking chopper/LConn1
  Measures/RConn1 -- Permanent Magnet Synchronous Machine/LConn1
  Measures/RConn2 -- Permanent Magnet Synchronous Machine/LConn2
  Measures/RConn3 -- Permanent Magnet Synchronous Machine/LConn3
  Measures/LConn1 -- Three-phase Inverter/RConn1
  Measures/LConn2 -- Three-phase Inverter/RConn2
  Measures/LConn3 -- Three-phase Inverter/RConn3

== system Main_simulation_optimised_accel_testbed/Sensing/demux ==
  motor : Inport
  Conv. : Inport  Port=2
  Ctrl : Inport  Port=3
  Bus Selector : BusSelector  OutputSignals=Stator current is_a (A),Rotor speed wm (rad/s),Electromagnetic torque Te (N*m)
  Bus Selector1 : BusSelector  OutputSignals=Torque reference (Nm),Reference
  Bus Selector2 : BusSelector  OutputSignals=V bus (V)
  Gain : Gain  Gain=30/pi  SaturateOnIntegerOverflow=on  OutDataTypeStr=Inherit: Same as input  ParamDataTypeStr=Inherit: Same as input
  Mux : Mux  Inputs=2
  Mux1 : Mux  Inputs=2
  i_a : Outport
  speed : Outport  Port=2
  Tem : Outport  Port=3
  v_dc : Outport  Port=4
  wires:
  Bus Selector/2 -> Gain/1  "<Rotor speed wm (rad/s)>"
  Bus Selector2/1 -> v_dc/1  "<V bus (V)>"
  Conv./1 -> Bus Selector2/1
  Ctrl/1 -> Bus Selector1/1
  Bus Selector1/1 -> Mux1/2  "<Torque reference (Nm)>"
  Bus Selector1/2 -> Mux/2  "<Reference>"
  Gain/1 -> Mux/1
  Bus Selector/1 -> i_a/1  "<Stator current is_a (A)>"
  Bus Selector/3 -> Mux1/1  "<Electromagnetic torque Te (N*m)>"
  Mux1/1 -> Tem/1
  Mux/1 -> speed/1
  motor/1 -> Bus Selector/1

== system Main_simulation_optimised_accel_testbed/Temperature/Motor_Temp_Subsys ==
  note: MOTOR TEMPERATURE
  note: for motor current of 20 amps peak, rms = 14.14A => i^2 = 200Watts of heat
      |  but with passive cooling the temperature and due to self radiative cooling the
      | temp is lower. Thus thermal coeff is set to 0.25, nominally the motor faces 20watts of withheld heat
  DRMS : sdolib/RMS Blocks/DRMS  Ts=1e-6
      settings: SourceProductName=Simulink Design Optimization  SourceProductBaseCode=SO
  Gain : Gain  Gain=0.01
  Math Function : Math  Operator=square  SaturateOnIntegerOverflow=on
  Math Function1 : Math  SaturateOnIntegerOverflow=on
  Rate Limiter : RateLimiter  SampleTimeMode=inherited
  Saturation2 : Saturate  UpperLimit=0  LowerLimit=-10
  Selector : Selector  InputPortWidth=3  IndexOptions=Index vector (dialog)  Indices=[1]  OutputSizes=1
  Subtract1 : Sum  Inputs=++++
  ambient : Constant  Value=25
  thermal coeff : Gain  Gain=2
  Out1 : Outport
  motor_temp(C) : Outport  Port=2
  tag scope: motor_temp=global
  wires:
  [iabcSens] -> Selector/1
  Selector/1 -> DRMS/1
  Math Function/1 -> thermal coeff/1
  DRMS/1 -> Math Function/1
  Rate Limiter/1 -> Subtract1/3
  Math Function1/1 -> Rate Limiter/1
  ambient/1 -> Out1/1
  Saturation2/1 -> Subtract1/4
  [speed_rpm] -> Gain/1
  Gain/1 -> Math Function1/1
  thermal coeff/1 -> Subtract1/2
  [temp_amb] -> Subtract1/1
  [cooling_rate] -> Saturation2/1
  Subtract1/1 -> motor_temp(C)/1, [motor_temp]  "motor_temp(C)"

== system Main_simulation_optimised_accel_testbed/Ultra Capacitor Subsys 200F1/UC_energy_monitor ==
  UC_power : Inport
  Constant : Constant  Value=0
  Discrete-Time Integrator : DiscreteIntegrator  InitialConditionSetting=State (most efficient)  SampleTime=-1  ICPrevOutput=DiscIntNeverNeededParam  ICPrevScaledInput=DiscIntNeverNeededParam
  Discrete-Time Integrator1 : DiscreteIntegrator  InitialConditionSetting=State (most efficient)  SampleTime=-1  ICPrevOutput=DiscIntNeverNeededParam  ICPrevScaledInput=DiscIntNeverNeededParam
  Relational Operator : RelationalOperator  Operator=>  OutDataTypeStr=boolean  RndMeth=Simplest
  Relational Operator1 : RelationalOperator  Operator=<  OutDataTypeStr=boolean  RndMeth=Simplest
  power_in : Product
  power_out : Product
  energy_out_UC : Outport
  energy_in_UC : Outport  Port=2
  wires:
  Constant/1 -> Relational Operator1/2, Relational Operator/2
  power_out/1 -> Discrete-Time Integrator/1
  power_in/1 -> Discrete-Time Integrator1/1
  Relational Operator1/1 -> power_in/1
  Discrete-Time Integrator/1 -> energy_out_UC/1  "energy_out_UC"
  Discrete-Time Integrator1/1 -> energy_in_UC/1  "energy_in_UC"
  UC_power/1 -> Relational Operator/1, Relational Operator1/1, power_in/2, power_out/2
  Relational Operator/1 -> power_out/1
